simulink model "Simulation"  (R2020b)
settings: Solver=VariableStepAuto  StartTime=0.0  StopTime=20  RelTol=1e-3
undefined symbols (not defined in the file or in its folder): DiscIntNeverNeededParam
libraries: mpclib x1, Library x1, sharedtransform x1
settings Model: Creator=keati  LastModifiedBy=keati

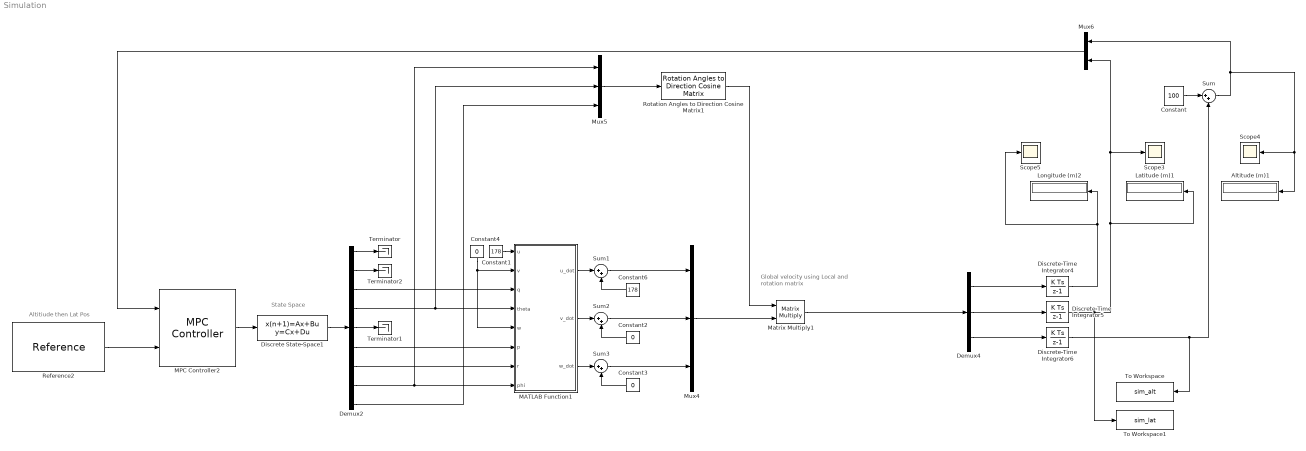
== system Simulation ==
  note: Global velocity using
      | Local and rotation
      | matrix
  note: Altitiude then Lat Pos
  note: State Space
  Altitude (m)1 : Display
  Constant : Constant  Value=100
  Constant1 : Constant  Value=178
  Constant2 : Constant  Value=0
  Constant3 : Constant  Value=0
  Constant4 : Constant  Value=0
  Constant6 : Constant  Value=178
  Demux2 : Demux  Outputs=9
  Demux4 : Demux  Outputs=3
  Discrete State-Space1 : DiscreteStateSpace  A=|  B=|  C=|  D=|  SampleTime=-1
      A=|
      | [1.0000    0.0001   -0.2905   -0.0968         0         0         0         0         0;
      |    -0.0007    0.9970    1.7422   -0.0159         0         0         0         0         0;
      |     0.0000   -0.0001    0.9955    0.0000         0         0         0         0         0;
      |     0.0000   -0.0000    0.0100    1.0000         0         0         0         0         0;
      |          0         0         0         0    0.9993    0.2901   -1.7547    0.0968    0.0160;
      |          0         0         0         0   -0.0006    0.9920   -0.0025   -0.0000   -0.0000;
      |          0         0         0         0    0.0001   -0.0002    0.9986    0.0000    0.0000;
      |          0         0         0         0   -0.0000    0.0100   -0.0000    1.0000   -0.0000;
      |          0         0         0         0    0.0000   -0.0000    0.0100    0.0000    1.0000];
      B=|
      | [0.0175         0         0;
      |    -0.1055         0         0;
      |    -0.0488         0         0;
      |    -0.0002         0         0;
      |          0    0.0034    0.0331;
      |          0    0.0468    0.0077;
      |          0    0.0009   -0.0136;
      |          0    0.0002    0.0000;
      |          0    0.0000   -0.0001];
      C=|
      | [1     0     0     0     0     0     0     0     0;
      |      0     1     0     0     0     0     0     0     0;
      |      0     0     1     0     0     0     0     0     0;
      |      0     0     0     1     0     0     0     0     0;
      |      0     0     0     0     1     0     0     0     0;
      |      0     0     0     0     0     1     0     0     0;
      |      0     0     0     0     0     0     1     0     0;
      |      0     0     0     0     0     0     0     1     0;
      |      0     0     0     0     0     0     0     0     1];
      D=|
      | [0     0     0;
      |      0     0     0;
      |      0     0     0;
      |      0     0     0;
      |      0     0     0;
      |      0     0     0;
      |      0     0     0;
      |      0     0     0;
      |      0     0     0];
  Discrete-Time Integrator4 : DiscreteIntegrator  SampleTime=-1  ICPrevOutput=DiscIntNeverNeededParam  ICPrevScaledInput=DiscIntNeverNeededParam
  Discrete-Time Integrator5 : DiscreteIntegrator  SampleTime=-1  ICPrevOutput=DiscIntNeverNeededParam  ICPrevScaledInput=DiscIntNeverNeededParam
  Discrete-Time Integrator6 : DiscreteIntegrator  SampleTime=-1  ICPrevOutput=DiscIntNeverNeededParam  ICPrevScaledInput=DiscIntNeverNeededParam
  Latitude (m)1 : Display
  Longitude (m)2 : Display
  MATLAB Function1 : MATLAB Function  TreatAsAtomicUnit=on
  MPC Controller2 : mpclib/MPC Controller  SCDEnableBlockLinearizationSpecification=on  mpcobj=mpc1  is_multiple=0  enable_value=0  return_u0=off  updateMPCinCallerWorkspace=on  md_inport=off  mv_inport=off  uref_inport=off  return_cost=off  return_mvseq=off  return_qpstatus=off  return_xseq=off  return_state=off  return_ovseq=off  state_inport=off  umin_inport=off  umax_inport=off  ymin_inport=off  ymax_inport=off  cc_inport=off  ywt_inport=off  uwt_inport=off  duwt_inport=off  rhoeps_inport=off  pm_inport=off  MaximumP=10  HorizonChoice=FixedHorizon  n_ts=0.01  n_p=100  n_mv=3  n_md=0  n_ud=0  n_mo=2  n_uo=0  BlockDataType=double  SampleTimeInherited=off  switch_inport=off
  Matrix Multiply1 : Product  Multiplication=Matrix(*)
  Mux4 : Mux  Inputs=3
  Mux5 : Mux  Inputs=3
  Mux6 : Mux  Inputs=2
  Reference2 : Library/Reference  SystemSampleTime=-1  VariantActivationTime=update diagram  Latency=0  AutoFrameSizeCalculation=off
  Rotation Angles to Direction Cosine Matrix1 : sharedtransform/Rotation Angles to Direction Cosine Matrix  rotationOrder=ZYX  aMode=aMode
      settings: SourceProductBaseCode=AE,PW,MT,UV,VE,VP
  Scope3 : Scope
  Scope4 : Scope
  Scope5 : Scope
  Sum{,1..3} (4 alike) : Sum  Inputs=|++
  Terminator : Terminator
  Terminator1 : Terminator
  Terminator2 : Terminator
  To Workspace : ToWorkspace  VariableName=sim_alt  SampleTime=-1
  To Workspace1 : ToWorkspace  VariableName=sim_lat  SampleTime=-1
  wires:
  Mux6/1 -> MPC Controller2/1
  Demux2/4 -> MATLAB Function1/4(theta), Mux5/2
  Demux2/7 -> MATLAB Function1/7(r)
  Rotation Angles to Direction Cosine Matrix1/1 -> Matrix Multiply1/1
  Discrete State-Space1/1 -> Demux2/1
  Mux4/1 -> Matrix Multiply1/2
  Demux4/1 -> Discrete-Time Integrator4/1
  MPC Controller2/1 -> Discrete State-Space1/1
  Reference2/1 -> MPC Controller2/2
  Demux4/3 -> Discrete-Time Integrator6/1
  Matrix Multiply1/1 -> Demux4/1
  Discrete-Time Integrator4/1 -> Longitude (m)2/1, Scope5/1
  Demux2/6 -> MATLAB Function1/6(p)
  Demux2/8 -> MATLAB Function1/8(phi), Mux5/1
  Demux2/3 -> MATLAB Function1/3(q)
  Demux4/2 -> Discrete-Time Integrator5/1
  Discrete-Time Integrator5/1 -> To Workspace1/1, Scope3/1, Mux6/2, Latitude (m)1/1
  Demux2/1 -> Terminator/1
  Demux2/2 -> Terminator2/1
  Demux2/5 -> Terminator1/1
  Constant2/1 -> Sum2/2
  Constant3/1 -> Sum3/2
  Sum3/1 -> Mux4/3
  Sum2/1 -> Mux4/2
  Sum1/1 -> Mux4/1
  MATLAB Function1/3(w_dot) -> Sum3/1
  MATLAB Function1/2(v_dot) -> Sum2/1
  MATLAB Function1/1(u_dot) -> Sum1/1
  Constant6/1 -> Sum1/2
  Constant1/1 -> MATLAB Function1/1(u)
  Constant4/1 -> MATLAB Function1/5(w), MATLAB Function1/2(v)
  Mux5/1 -> Rotation Angles to Direction Cosine Matrix1/1
  Demux2/9 -> Mux5/3
  Discrete-Time Integrator6/1 -> To Workspace/1, Sum/2
  Sum/1 -> Scope4/1, Altitude (m)1/1, Mux6/1
  Constant/1 -> Sum/1

== matlab function Simulation/MATLAB Function1 ==
  data: u input; v input; q input; theta input; w input; p input; r input; phi input; u_dot output; v_dot output; w_dot output
function [u_dot, v_dot, w_dot] = fcn(u, v, q, theta, w,  p, r, phi )

X = 18825*0.86 - ((.047*.3809*178^2*49.239)/2) / 8.58; % thrust - drag 
Z = (.047*.3809*178^2*49.239) / 2 - 18825;% lift - weight
Y =  Z*sin(-.005078); % lateral force

u_dot = (X/17642 - 9.81*sin(theta) + r*v - q*w )*.01;

v_dot = (Y/17642 - 9.81*sin(phi)*cos(theta) - r*u + q*w)*.01 ;

w_dot = (Z/17642 - 9.81*cos(phi)*cos(theta) - q*u - p*v)*.01 ;
